simulink model "PIDzn"  (R2020a)
settings: Solver=VariableStepAuto  StartTime=0.0  StopTime=20  RelTol=1e-5
settings Model: Creator=batis  LastModifiedBy=batis

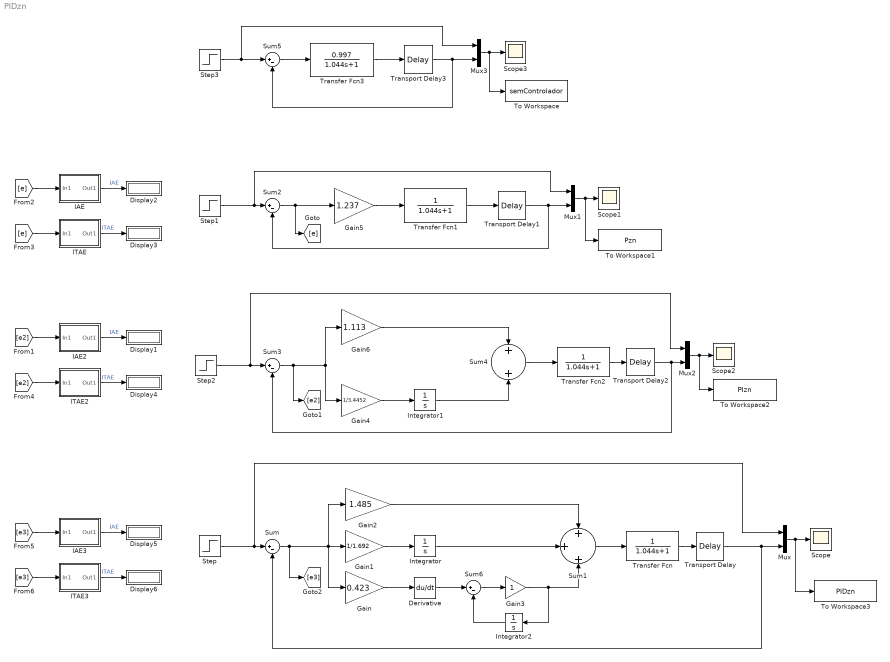
== system PIDzn ==
  Derivative : Derivative
  Display{1..6} (6 alike) : Display
  Gain : Gain  Gain=0.423
  Gain1 : Gain  Gain=1/1.692
  Gain2 : Gain  Gain=1.485
  Gain3 : Gain
  Gain4 : Gain  Gain=1/3.4452
  Gain5 : Gain  Gain=1.237
  Gain6 : Gain  Gain=1.113
  IAE : Subsystem
  IAE2 : Subsystem
  IAE3 : Subsystem
  ITAE : Subsystem
  ITAE2 : Subsystem
  ITAE3 : Subsystem
  Integrator : Integrator
  Integrator1 : Integrator
  Integrator2 : Integrator
  Mux{,1..3} (4 alike) : Mux  Inputs=2
  Scope{,1..3} (4 alike) : Scope
  Step{,1..3} (4 alike) : Step  After=3  SampleTime=0
  Sum{,2..3,5..6} (5 alike) : Sum  Inputs=|+-
  Sum1 : Sum  Inputs=+|+|+
  Sum4 : Sum  Inputs=+|+
  To Workspace : ToWorkspace  VariableName=semControlador  SaveFormat=Structure With Time  SampleTime=-1
  To Workspace1 : ToWorkspace  VariableName=Pzn  SaveFormat=Structure With Time  SampleTime=-1
  To Workspace2 : ToWorkspace  VariableName=PIzn  SaveFormat=Structure With Time  SampleTime=-1
  To Workspace3 : ToWorkspace  VariableName=PIDzn  SaveFormat=Structure With Time  SampleTime=-1
  Transfer Fcn : TransferFcn  Denominator=[1.044 1]
  Transfer Fcn1 : TransferFcn  Denominator=[1.044 1]
  Transfer Fcn2 : TransferFcn  Denominator=[1.044 1]
  Transfer Fcn3 : TransferFcn  Numerator=[0.997]  Denominator=[1.044 1]
  Transport Delay : TransportDelay  DelayTime=0.846
  Transport Delay1 : TransportDelay  DelayTime=0.846  FixedBuffer=on
  Transport Delay2 : TransportDelay  DelayTime=0.846
  Transport Delay3 : TransportDelay  DelayTime=0.846  FixedBuffer=on
  wires:
  Sum/1 -> [e3], Gain/1, Gain2/1, Gain1/1
  Sum1/1 -> Transfer Fcn/1
  Step/1 -> Sum/1, Mux/1
  Mux/1 -> To Workspace3/1, Scope/1
  Gain/1 -> Derivative/1
  Transfer Fcn/1 -> Transport Delay/1
  Transport Delay/1 -> Sum/2, Mux/2
  Gain2/1 -> Sum1/1
  Gain1/1 -> Integrator/1
  Integrator/1 -> Sum1/2
  Mux1/1 -> To Workspace1/1, Scope1/1
  Sum2/1 -> [e], Gain5/1
  Gain5/1 -> Transfer Fcn1/1
  Step1/1 -> Sum2/1, Mux1/1
  Transfer Fcn1/1 -> Transport Delay1/1
  Transport Delay1/1 -> Mux1/2, Sum2/2
  Gain6/1 -> Sum4/1
  Transport Delay2/1 -> Mux2/2, Sum3/2
  Mux2/1 -> To Workspace2/1, Scope2/1
  Sum3/1 -> [e2], Gain6/1, Gain4/1
  Gain4/1 -> Integrator1/1
  Transfer Fcn2/1 -> Transport Delay2/1
  Integrator1/1 -> Sum4/2
  Sum4/1 -> Transfer Fcn2/1
  Step2/1 -> Mux2/1, Sum3/1
  Transport Delay3/1 -> Mux3/2, Sum5/2
  Step3/1 -> Sum5/1, Mux3/1
  Transfer Fcn3/1 -> Transport Delay3/1
  Mux3/1 -> To Workspace/1, Scope3/1
  Sum5/1 -> Transfer Fcn3/1
  Derivative/1 -> Sum6/1
  Sum6/1 -> Gain3/1
  Gain3/1 -> Integrator2/1, Sum1/3
  Integrator2/1 -> Sum6/2
  [e3] -> IAE3/1(In1)
  [e] -> IAE/1(In1)
  [e3] -> ITAE3/1(In1)
  ITAE3/1(Out1) -> Display6/1  "ITAE"
  [e] -> ITAE/1(In1)
  ITAE/1(Out1) -> Display3/1  "ITAE"
  IAE/1(Out1) -> Display2/1  "IAE"
  [e2] -> IAE2/1(In1)
  [e2] -> ITAE2/1(In1)
  IAE2/1(Out1) -> Display1/1  "IAE"
  IAE3/1(Out1) -> Display5/1  "IAE"
  ITAE2/1(Out1) -> Display4/1  "ITAE"

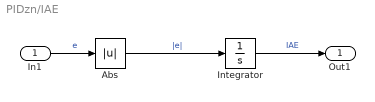
== system PIDzn/IAE ==
  In1 : Inport
  Abs : Abs
  Integrator : Integrator
  Out1 : Outport
  wires:
  Integrator/1 -> Out1/1  "IAE"
  In1/1 -> Abs/1  "e"
  Abs/1 -> Integrator/1  "|e|"

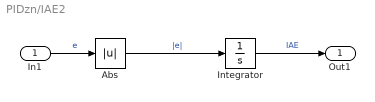
== system PIDzn/IAE2 ==
  In1 : Inport
  Abs : Abs
  Integrator : Integrator
  Out1 : Outport
  wires:
  Integrator/1 -> Out1/1  "IAE"
  In1/1 -> Abs/1  "e"
  Abs/1 -> Integrator/1  "|e|"

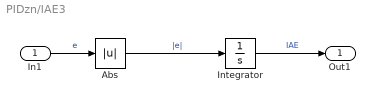
== system PIDzn/IAE3 ==
  In1 : Inport
  Abs : Abs
  Integrator : Integrator
  Out1 : Outport
  wires:
  Integrator/1 -> Out1/1  "IAE"
  In1/1 -> Abs/1  "e"
  Abs/1 -> Integrator/1  "|e|"

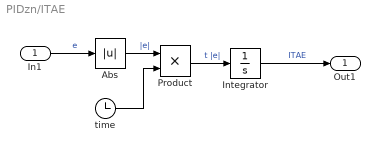
== system PIDzn/ITAE ==
  In1 : Inport
  Abs : Abs
  Integrator : Integrator
  Product : Product
  time : Clock
  Out1 : Outport
  wires:
  In1/1 -> Abs/1  "e"
  Integrator/1 -> Out1/1  "ITAE"
  time/1 -> Product/2
  Abs/1 -> Product/1  "|e|"
  Product/1 -> Integrator/1  "t |e|"

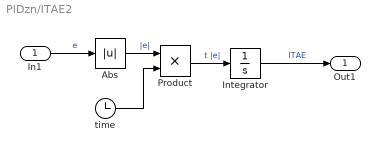
== system PIDzn/ITAE2 ==
  In1 : Inport
  Abs : Abs
  Integrator : Integrator
  Product : Product
  time : Clock
  Out1 : Outport
  wires:
  In1/1 -> Abs/1  "e"
  Integrator/1 -> Out1/1  "ITAE"
  time/1 -> Product/2
  Abs/1 -> Product/1  "|e|"
  Product/1 -> Integrator/1  "t |e|"

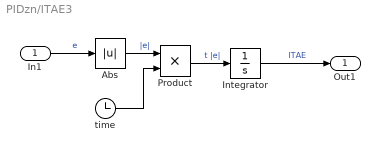
== system PIDzn/ITAE3 ==
  In1 : Inport
  Abs : Abs
  Integrator : Integrator
  Product : Product
  time : Clock
  Out1 : Outport
  wires:
  In1/1 -> Abs/1  "e"
  Integrator/1 -> Out1/1  "ITAE"
  time/1 -> Product/2
  Abs/1 -> Product/1  "|e|"
  Product/1 -> Integrator/1  "t |e|"
